simulink model "tv_controller_"  (R2023a)
settings: Solver=VariableStepAuto  StartTime=0.0  StopTime=10.0  RelTol=1e-3
values from neighbouring files (symbols this model uses):
  GCoSim_Name = 'GCoSim1'    [car_ver1_GCoSim1.m]    (also in car_ver1_GCoSim2.m = 'GCoSim2'; pure_GCoSim1.m)
  GCoSim_Name_n = r_temp___(2)    [car_ver1_GCoSim1.m]    (also in car_ver1_GCoSim2.m; pure_GCoSim1.m)
  Matlab_version = str2double(splited_Version__(1))    [car_ver1_GCoSim1.m]    (also in car_ver1_GCoSim2.m; pure_GCoSim1.m)
  Output_File = 'car_ver1_GCoSim1'    [car_ver1_GCoSim1.m]    (also in car_ver1_GCoSim2.m = 'car_ver1_GCoSimulink_GCoSim2'; pure_GCoSim1.m = 'pure_GCoSim1')
  Output_file_n = r_temp___(2)    [car_ver1_GCoSim1.m]    (also in car_ver1_GCoSim2.m; pure_GCoSim1.m)
  Plant_inputs_num = r_temp___(1)    [car_ver1_GCoSim1.m]    (also in car_ver1_GCoSim2.m; pure_GCoSim1.m)
  Plant_outputs_num = r_temp___(1)    [car_ver1_GCoSim1.m]    (also in car_ver1_GCoSim2.m; pure_GCoSim1.m)
  RecurDyn = 'C:\Program Files\FunctionBay, Inc\RecurDyn 2024\Bin\'    [car_ver1_GCoSim1.m]    (also in car_ver1_GCoSim2.m; pure_GCoSim1.m)
  RecurDyn_controltimestep = 1.e-003    (= 0.001)    [car_ver1_GCoSim1.m]    (also in car_ver1_GCoSim2.m; pure_GCoSim1.m)
  RecurDyn_model = 'car_ver1.rdyn'    [car_ver1_GCoSim1.m]    (also in car_ver1_GCoSim2.m; pure_GCoSim1.m = 'pure.rdyn')
  RecurDyn_model_n = r_temp___(2)    [car_ver1_GCoSim1.m]    (also in car_ver1_GCoSim2.m; pure_GCoSim1.m)
settings Model: Creator=Dell  LastModifiedBy=kgt22
settings RTWCC: GPUComputeCapability=5.0

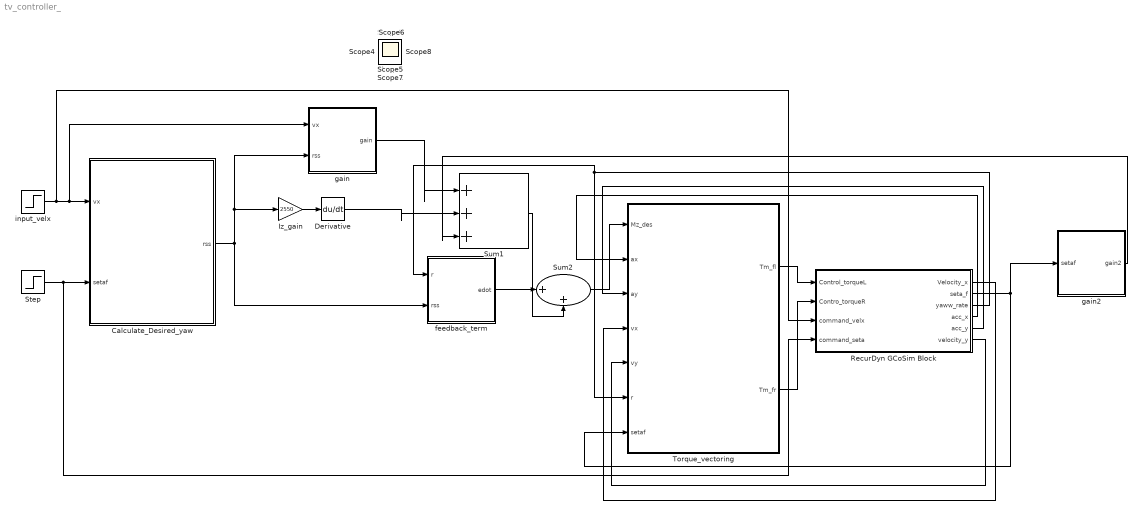
== system tv_controller_ ==
  Calculate_Desired_yaw : MATLAB Function  TreatAsAtomicUnit=on
  Derivative : Derivative
  Iz_gain : Gain  Gain=2550
  RecurDyn GCoSim Block : Subsystem
      mask Display: image(imread('RecurDyn_GCoSimIF_Host.png'))
  Step : Step  Time=0.1  Before=0.00  After=0.05  SampleTime=10
  Sum1 : Sum  Inputs=|+++
  Sum2 : Sum  Inputs=|++
  Torque_vectoring : MATLAB Function  TreatAsAtomicUnit=on
  feedback_term : MATLAB Function  TreatAsAtomicUnit=on
  gain : MATLAB Function  TreatAsAtomicUnit=on
  gain2 : MATLAB Function  TreatAsAtomicUnit=on
  input_velx : Step  Before=15  After=20  SampleTime=10
  Scope{,1..8} (9 alike) : Scope
  wires:
  Calculate_Desired_yaw/1(rss) -> feedback_term/2(rss), Iz_gain/1, gain/2(rss)
  input_velx/1 -> RecurDyn GCoSim Block/3("command_velx   "), gain/1(vx), Calculate_Desired_yaw/1(vx)
  gain/1(gain) -> Sum1/1
  Derivative/1 -> Sum1/2
  RecurDyn GCoSim Block/2("seta_f    ") -> gain2/1(setaf), Torque_vectoring/7(setaf)
  gain2/1(gain2) -> Sum1/3
  Sum1/1 -> Sum2/2
  RecurDyn GCoSim Block/3("yaww_rate ") -> feedback_term/1(r), Torque_vectoring/6(r)
  feedback_term/1(edot) -> Sum2/1
  Torque_vectoring/1(Tm_fl) -> RecurDyn GCoSim Block/1(Control_torqueL)
  Torque_vectoring/2(Tm_fr) -> RecurDyn GCoSim Block/2("Contro_torqueR ")
  Sum2/1 -> Torque_vectoring/1(Mz_des)
  RecurDyn GCoSim Block/4("acc_x     ") -> Torque_vectoring/2(ax)
  RecurDyn GCoSim Block/5("acc_y     ") -> Torque_vectoring/3(ay)
  RecurDyn GCoSim Block/1(Velocity_x) -> Torque_vectoring/4(vx)
  RecurDyn GCoSim Block/6(velocity_y) -> Torque_vectoring/5(vy)
  Step/1 -> RecurDyn GCoSim Block/4("command_seta   "), Calculate_Desired_yaw/2(setaf)
  Iz_gain/1 -> Derivative/1

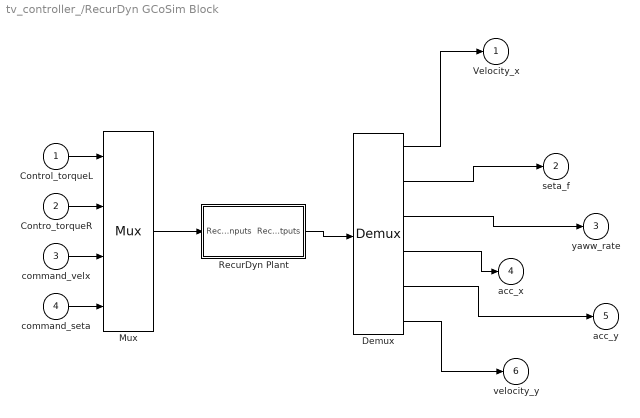
== system tv_controller_/RecurDyn GCoSim Block ==
  Control_torqueL : Inport
  "Contro_torqueR " : Inport  Port=2
  "command_velx   " : Inport  Port=3
  "command_seta   " : Inport  Port=4
  Demux : Demux  Outputs=6
      settings: DisplayOption=none
  Mux : Mux
  RecurDyn Plant : Subsystem  mask(Recurdyn/Plant){RecurDyn_model_name=RecurDyn_model, GCoSim_Name_=GCoSim_Name, Output_File_Name_=Output_File, RecurDyn_=RecurDyn, Matlab_version_=Matlab_version, RecurDyn_controltimestep_=RecurDyn_controltimestep, RecurDyn_step_=100, Waitingtime=1000, RecurDyn_static_=off, RecurDyn_show_=on, RecurDyn_ani_=on, Create_Output_Folder_=off}
      mask prompts: GCoSim_Name_ "GCoSim Name"; Output_File_Name_ "Output File Name"; RecurDyn_ "RecurDyn_install_directory"; Matlab_version_ "Matlab version"; RecurDyn_controltimestep_ "Sampling period"; RecurDyn_step_ "RecurDyn_step"; Waitingtime "Waiting time"; RecurDyn_static_ "Static analysis"; RecurDyn_show_ "RecurDyn_show"; RecurDyn_ani_ "RecurDyn_animation"; Create_Output_Folder_ "Create Output Folder"
      mask help:
      | This block is able to simulate for any Recurdyn Dynamics Model as Recurdyn/GCoSim Solver.
      | All Data of Plant inputs/outputs are transfered at every sampling time which is defined by Sampling Period (Control Time Step).
      mask Display: disp( 'Dynamic Model' )
  Velocity_x : Outport
  "seta_f    " : Outport  Port=2
  "yaww_rate " : Outport  Port=3
  "acc_x     " : Outport  Port=4
  "acc_y     " : Outport  Port=5
  velocity_y : Outport  Port=6
  wires:
  "command_seta   "/1 -> Mux/4
  "command_velx   "/1 -> Mux/3
  "Contro_torqueR "/1 -> Mux/2
  Control_torqueL/1 -> Mux/1
  Demux/6 -> velocity_y/1
  Demux/5 -> "acc_y     "/1
  Demux/4 -> "acc_x     "/1
  Demux/3 -> "yaww_rate "/1
  Demux/2 -> "seta_f    "/1
  Demux/1 -> Velocity_x/1
  Mux/1 -> RecurDyn Plant/1(" RecurDyn_inputs")
  RecurDyn Plant/1(RecurDyn_outputs) -> Demux/1

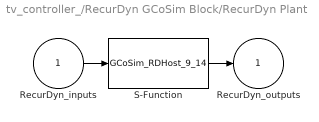
== system tv_controller_/RecurDyn GCoSim Block/RecurDyn Plant ==
  " RecurDyn_inputs" : Inport
  S-Function : S-Function  FunctionName=GCoSim_RDHost_9_14  Parameters=RecurDyn_controltimestep_,RecurDyn_model_name,RecurDyn_,RecurDyn_static_,RecurDyn_step_,RecurDyn_show_,RecurDyn_ani_,Matlab_version_,RecurDyn_model_n,Plant_inputs_num,Plant_outputs_num,Waitingtime,Create_Output_Folder_,Output_File_Name_,Output_file_n,GCoSim_Name_,GCoSim_Name_n  SFunctionDeploymentMode=off  EnableBusSupport=off
  RecurDyn_outputs : Outport  InitialOutput=0  VectorParamsAs1DForOutWhenUnconnected=off
  wires:
  " RecurDyn_inputs"/1 -> S-Function/1
  S-Function/1 -> RecurDyn_outputs/1

== matlab function tv_controller_/Calculate_Desired_yaw ==
  data: rss output; vx input; setaf input
function rss   = dyn_model (vx, setaf)

Kv = 1.034e-003;
L = 2746.83;

r = vx/(L + Kv*vx^2);
rss = r * setaf;

== matlab function tv_controller_/gain ==
  data: gain output; vx input; rss input
function gain   = dyn_model (vx,rss)

Cf = 500000; %500009
Cr = 500000;
Lf = 900;
Lr = 1846.83;

gai = (Cf*Lf^2 + Cr*Lr^2);
gai2 = gai / vx;
gain = rss * gai2;

== matlab function tv_controller_/gain2 ==
  data: gain2 output; setaf input
function gain2   = dyn_model (setaf)

Cf = 500009;
Lf = 900;

gain2 = - setaf * Cf*Lf;

== matlab function tv_controller_/feedback_term ==
  data: edot output; r input; rss input
function edot   = sat_e (r, rss)

positive_proportional_gain = 0.62;
e = r - rss;
pos_sat_boundary = 1; %이부분 정확하게

if pos_sat_boundary<e
    sat_e = 1;
elseif e < -pos_sat_boundary
    sat_e = -1;
else
    sat_e = e / pos_sat_boundary;
end

edot = -positive_proportional_gain * sat_e;

== matlab function tv_controller_/Torque_vectoring ==
  data: Tm_fl output; Mz_des input; Tm_fr output; ax input; ay input; vx input; vy input; r input; setaf input
function [ Tm_fl, Tm_fr ] = Torque_distribution (Mz_des , ax, ay,vx,vy, r, setaf )
m = 1500; % kg
g = 9.81; % m/s^2
L = 2746.83;
Lf = 900;
Lr = 1846.83;
h = 300; % height of CG, mm
Iz = 2550000000;
t = 1600; %track width
Re = 335 % Effective tire radius, mm
Cf = 500000; %N/rad 실제 차아님 논문참
Cr = 500000;

beta = vy/vx % for very small angle

% rdot z모멘트로 계산
rdot = (Cr*Lr - Cf*Lf)*beta / Iz - (Cf*Lf^2 + Cr*Lr^2)*r / (Iz*vx) + (Cf*Lf*setaf) / Iz; %Mz / Iz 외란이라 생각하고 제거

%최대 토크 구하기 위한 수직, 횡력 구하기
Fz_fl = m*g*Lr/(2*L) - m*h*ax/(2*L) - m*h*ay;
Fz_fr =  m*g*Lr/(2*L) - m*h*ax/(2*L) + m*h*ay;

Fyf = (m*Lr*ay + Iz*rdot - Mz_des)/L;

% for get F_ratio = Fy_fl/Fy_fr 
nominator = (vx*beta + r*Lf) / (vx - r*t/2) - setaf;
denominator = (vx*beta + r*Lf) / (vx + r*t/2) - setaf;
F_ratio = (Fz_fl / Fz_fr) * nominator / denominator;
if F_ratio >1
    F_ratio = 1;
elseif F_ratio <0
    F_ratio = 0;
end

Fy_fl = Fyf / ( 1 + 1/F_ratio);
Fy_fr = Fyf / (1 + F_ratio);


Tm_max_fl = iwm_torque_friction(Fz_fl,Fy_fl);
Tm_max_fr = iwm_torque_friction(Fz_fr,Fy_fr);
% T-N curve에서의 최대 토크값과 비교해 min을 해야 하지만, 시뮬레이션이라 일단

Tm_reg_max = 200; % 토크 regulator max값 (정규 상수, 논문 200Nm)
% fl, fr 두개잇는데 차이는모르겠

if Mz_des >=0
    Mz_lim = t*(Tm_max_fr - Tm_reg_max)/(2*Re);
else
    Mz_lim = t*(Tm_max_fl - Tm_reg_max)/(2*Re);
end

%계산된 최대 모멘트, desired 모멘트로 토크 분배
alpha = 0.5 %(0<=alpha<=1),  By adjusting 𝛼, it is possible to freely tune the timing of the negative IWM torque intervention

if Mz_des < -alpha*Mz_lim
    Tm_fl = Re*(alpha*Mz_lim - Mz_des) / t
elseif Mz_des <0
    Tm_fl = -2*Re*Mz_des; %여기 Mz_des_f라 되있는데 오탄가..?
elseif Mz_des <=alpha*Mz_lim
    Tm_fl = 0
else
    Tm_fl = Re*(alpha * Mz_lim - Mz_des) / t;
end

if Mz_des < -alpha*Mz_lim
    Tm_fr = Re*(alpha*Mz_lim + Mz_des) / t
elseif Mz_des <0
    Tm_fr = 0;
elseif Mz_des <=alpha*Mz_lim
    Tm_fr = 2*Re*Mz_des;
else
    Tm_fr = Re*(alpha * Mz_lim + Mz_des) / t;
end




%get T_m_max_i 최대 토크
function friction_circle = iwm_torque_friction(Fz , Fy)
Re = 335; %effective tire radius (mm)
u = 1.1; % tire friction
friction_circle = Re * sqrt(abs(u^2 * Fz ^2 - Fy^2))
